simulink model "BlueROV2_Exp_Simu_NIF"  (R2023b)
settings: Solver=FixedStepAuto  StartTime=0.0  StopTime=120  FixedStep=dt  RelTol=1e-3
values from neighbouring files (symbols this model uses):
  Af = diag(ti)    [RM_param_AGF.m]
  Ballast_Force = Ballast_Compute(Ballast_Config)    [Integrate.m]    (also in init.m = Ballast_Term(Ballast_Config); init_NIF.m = [0; 0; Ballast_Term; 0]; init_NIF2.m = [0; 0; Ballast_Term; 0]; init_ODE.m)
  dt = 0.1    [Integrate.m]    (also in init.m; init_NIF.m; init_NIF2.m; init_ODE.m)
  Gamma = diag(omega_is)    [RM_param_AGF.m]
  Kd = [155; 355; 8985; 1205; 1205; 1]    [Integrate.m]    (also in init.m = [1; 1; 1; 1; 1; 1]; init_NIF.m; init_NIF2.m; init_ODE.m)
  Ki = [45; 45; 10; 96; 96; 1]    [Integrate.m]    (also in init.m = [1; 1; 1; 1; 1; 1]; init_NIF.m; init_NIF2.m; init_ODE.m)
  Kp = [255; 545; 7095; 2420; 2375; 1]    [Integrate.m]    (also in init.m = [1; 1; 1; 1; 1; 1]; init_NIF.m; init_NIF2.m; init_ODE.m)
  lower_limit = -upper_limit    (= -30)    [Integrate.m]    (also in init.m; init_NIF.m; init_NIF2.m; init_ODE.m)
  Omega = diag(2*omega_is.*zeta_is)    [RM_param_AGF.m]
  Param = BlueROV2_param()    [Integrate.m]    (also in init.m; init_NIF.m; init_NIF2.m; init_ODE.m)
  T_alloc = Thrust_Allocation()    [Integrate.m]    (also in init_NIF.m; init_NIF2.m; init_ODE.m; init_ballast_checking.m)
  T_alloc_ps = pinv(T_alloc' * T_alloc + lambda * eye(size(T_alloc, 2))) * T_alloc'    [Integrate.m]    (also in init_NIF.m; init_NIF2.m; init_ODE.m; init_ballast_checking.m)
  thrust_rate = 5    [Integrate.m]    (also in init.m; init_NIF.m; init_NIF2.m; init_ODE.m)
  upper_limit = 30    [Integrate.m]    (also in init.m; init_NIF.m; init_NIF2.m; init_ODE.m)
undefined symbols (not defined in the file or in its folder): model_val, Phi_ref, Psi_ref, resampled_time, Theta_ref, time_stamps_phi, time_stamps_psi, time_stamps_theta, time_stamps_x, time_stamps_y, time_stamps_z, time_val, X_ref, Y_ref, Z_ref
(part 2 of 2)

== matlab function BlueROV2_Exp_Simu_NIF/Real Model/BlueROV2/BLUEROV2 DYNAMIC/ROV_SYSTEM/DYNAMIC SOLVER/BlueROV2_EOM/Nonlinear Damping ==
  data: F_nld_o output; nu_b input; d_CB input; K_nl input
function F_nld_o = Nonlinear_Damping_forces(nu_b, d_CB, K_nl)
%% Nonlinear Damping Forces
% Velocity
u = nu_b(1);
v = nu_b(2);
w = nu_b(3);
p = nu_b(4);
q = nu_b(5);
r = nu_b(6);

% Distance from CB to CO
% Defined as d_CB

% Transformed Velocity
V_t_b = H_(-d_CB) * nu_b;  % 6DOF Velocity, expressed in CB

% Nonlinear Damping Matrix
NL_Damping_Coeff = diag(K_nl) * abs(V_t_b);

% Force
F_nld_o = -(H_(d_CB))' * diag(NL_Damping_Coeff) * V_t_b;

% For debugging
% F_nld_o = -diag(NL_Damping_Coeff) * nu_b;
% F_nld_o = zeros(6,1);
end

== matlab function BlueROV2_Exp_Simu_NIF/Real Model/Reference Model CIF/Heave/MATLAB Function ==
  data: t input; eta_ref output; resampled_model input; resampled_time input
function eta_ref = feedPositionReference(t, resampled_model, resampled_time)
    persistent positionData;
    persistent timeData;
    persistent currentIndex;
    
    % Load position and time data (you can load this data only once)
    if isempty(positionData)
        positionData = resampled_model; % Your position data
        timeData = resampled_time; % Your time data
        currentIndex = 1;
    end
    
    % Find the index corresponding to the current time
    while currentIndex < length(timeData) && timeData(currentIndex) < t
        currentIndex = currentIndex + 1;
    end
    
    % Output the position reference at the current time
    eta_ref = positionData(currentIndex);
end

== matlab function BlueROV2_Exp_Simu_NIF/Real Model/Reference Model CIF/Pitch/MATLAB Function ==
  data: t input; eta_ref output; resampled_model input; resampled_time input
function eta_ref = feedPositionReference(t, resampled_model, resampled_time)
    persistent positionData;
    persistent timeData;
    persistent currentIndex;
    
    % Load position and time data (you can load this data only once)
    if isempty(positionData)
        positionData = resampled_model; % Your position data
        timeData = resampled_time; % Your time data
        currentIndex = 1;
    end
    
    % Find the index corresponding to the current time
    while currentIndex < length(timeData) && timeData(currentIndex) < t
        currentIndex = currentIndex + 1;
    end
    
    % Output the position reference at the current time
    eta_ref = positionData(currentIndex);
end

== matlab function BlueROV2_Exp_Simu_NIF/Real Model/Reference Model CIF/Roll/MATLAB Function ==
  data: t input; eta_ref output; resampled_model input; resampled_time input
function eta_ref = feedPositionReference(t, resampled_model, resampled_time)
    persistent positionData;
    persistent timeData;
    persistent currentIndex;
    
    % Load position and time data (you can load this data only once)
    if isempty(positionData)
        positionData = resampled_model; % Your position data
        timeData = resampled_time; % Your time data
        currentIndex = 1;
    end
    
    % Find the index corresponding to the current time
    while currentIndex < length(timeData) && timeData(currentIndex) < t
        currentIndex = currentIndex + 1;
    end
    
    % Output the position reference at the current time
    eta_ref = positionData(currentIndex);
end

== matlab function BlueROV2_Exp_Simu_NIF/Real Model/BlueROV2/BLUEROV2 DYNAMIC/ROV_SYSTEM/DYNAMIC SOLVER/Rotation Matrix ==
  data: eta_n input; J_Theta_nb output
function J_Theta_nb = Transform_nb(eta_n)
%%%%%%%%%%%%%%%%%%%%%%%%%%%%%%%%%%%%%%%%%%%%%%%%%%%%%%%%%%%%%%%%%%%%%%%%%%%
% Command                                                                 %
%                                                                         %
% Compute the Jacobian from {b} to {n}                                    %
%                                                                         %
% For 6-DOF Equations:                                                    %
% [ndot = Jacobian(n_theta) * v]                                          %
% -ndot = velocity expressed in NED frame                                 %
% -n_theta = rotational part of position vector                           %
% - v = velocity expressed in Body frame                                  %
%                                                                         %
% Argument:                                                               %
% eta     : Input positional vector                                       %
%                                                                         %
% Created:      27.09.2023	Andreas Sitorus                               %
%                                                                         %
%%%%%%%%%%%%%%%%%%%%%%%%%%%%%%%%%%%%%%%%%%%%%%%%%%%%%%%%%%%%%%%%%%%%%%%%%%%
%% Get the orientation
phi = eta_n(4,1);       % Rolling angle
theta = eta_n(5,1);     % Pitching angle
psi = eta_n(6,1);       % Yaw angle

%% Linear Velocity Transformation Matrix
% Element
r11 = cos(psi) * cos(theta);
r12 = -sin(psi) * cos(phi) + cos(psi) * sin(theta) * sin(phi);
r13 = sin(psi) * sin(phi) + cos(psi) * cos(phi) * sin(theta);
r21 = sin(psi) * cos(theta);
r22 = cos(psi) * cos(phi) + sin(phi) * sin(theta) * sin(psi);
r23 = -cos(psi) * sin(phi) + sin(theta) * sin(psi) * cos(phi);
r31 = -sin(theta);
r32 = cos(theta) * sin(phi);
r33 = cos(theta) * cos(phi);

% Rotation Matrix (from {b} to {n})
R_Theta_nb = [r11 r12 r13;
              r21 r22 r23;
              r31 r32 r33];

%% Angular Velocity Transformation Matrix
% Element
t11 = 1;
t12 = sin(phi) * tan(theta);
t13 = cos(phi) * tan(theta);
t21 = 0;
t22 = cos(phi);
t23 = -sin(phi);
t31 = 0;
t32 = sin(phi) / cos(theta);
t33 = cos(phi) / cos(theta);

% Angular Velocity Rotation Matrix (from {b} to {n})
T_Theta_nb = [t11 t12 t13;
              t21 t22 t23;
              t31 t32 t33];

%% Jacobian
J_Theta_nb = [R_Theta_nb  zeros(3);
              zeros(3) T_Theta_nb];

end

== matlab function BlueROV2_Exp_Simu_NIF/Real Model/Reference Model CIF/Surge/MATLAB Function ==
  data: t input; eta_ref output; resampled_model input; resampled_time input
function eta_ref = feedPositionReference(t, resampled_model, resampled_time)
    persistent positionData;
    persistent timeData;
    persistent currentIndex;
    
    % Load position and time data (you can load this data only once)
    if isempty(positionData)
        positionData = resampled_model; % Your position data
        timeData = resampled_time; % Your time data
        currentIndex = 1;
    end
    
    % Find the index corresponding to the current time
    while currentIndex < length(timeData) && timeData(currentIndex) < t
        currentIndex = currentIndex + 1;
    end
    
    % Output the position reference at the current time
    eta_ref = positionData(currentIndex);
end

== matlab function BlueROV2_Exp_Simu_NIF/Real Model/Reference Model CIF/Sway/MATLAB Function ==
  data: t input; eta_ref output; resampled_model input; resampled_time input
function eta_ref = feedPositionReference(t, resampled_model, resampled_time)
    persistent positionData;
    persistent timeData;
    persistent currentIndex;
    
    % Load position and time data (you can load this data only once)
    if isempty(positionData)
        positionData = resampled_model; % Your position data
        timeData = resampled_time; % Your time data
        currentIndex = 1;
    end
    
    % Find the index corresponding to the current time
    while currentIndex < length(timeData) && timeData(currentIndex) < t
        currentIndex = currentIndex + 1;
    end
    
    % Output the position reference at the current time
    eta_ref = positionData(currentIndex);
end

== matlab function BlueROV2_Exp_Simu_NIF/Real Model/Reference Model CIF/Yaw/MATLAB Function ==
  data: t input; eta_ref output; resampled_model input; resampled_time input
function eta_ref = feedPositionReference(t, resampled_model, resampled_time)
    persistent positionData;
    persistent timeData;
    persistent currentIndex;
    
    % Load position and time data (you can load this data only once)
    if isempty(positionData)
        positionData = resampled_model; % Your position data
        timeData = resampled_time; % Your time data
        currentIndex = 1;
    end
    
    % Find the index corresponding to the current time
    while currentIndex < length(timeData) && timeData(currentIndex) < t
        currentIndex = currentIndex + 1;
    end
    
    % Output the position reference at the current time
    eta_ref = positionData(currentIndex);
end

== matlab function BlueROV2_Exp_Simu_NIF/For Estimation/BlueROV2/BLUEROV2 DYNAMIC/ROV_SYSTEM/DYNAMIC SOLVER/BlueROV2_EOM/Added Mass Coriolis-Centripetal ==
  data: nu_b input; F_Ca_o output; d_CB input; AM input
function F_Ca_o    = Coriolis_Centripetal_AM_Force(nu_b, d_CB, AM)
%% Coriolis-Centripetal Forces
% Velocity
u = nu_b(1);
v = nu_b(2);
w = nu_b(3);
p = nu_b(4);
q = nu_b(5);
r = nu_b(6);

% Distance from CB to CO
% Defined as d_CB

% Transformed Velocity
V_t_b = H_(-d_CB) * nu_b;  % 6DOF Velocity, expressed in CB

% Added Mass Coefficient
Xud = AM(1);
Yvd = AM(2);
Zwd = AM(3);
Kpd = AM(4);
Mqd = AM(5);
Nrd = AM(6);

% CC-Added Mass
% Described in Body frame, at Center of Buoyancy
Ca11 = zeros(3);
Ca12 = [0 -Zwd*w Yvd*v;
        Zwd*w 0 -Xud*u;
        -Yvd*v Xud*u 0];
Ca21 = Ca12;
Ca22 = [0 -Nrd*r Mqd*q;
        Nrd*r 0 -Kpd*p;
        -Mqd*q Kpd*p 0];

Ca = [Ca11 Ca12;
      Ca21 Ca22]; % Added mass Coriolis Force Matrix, at Center of Buoyancy

% Force
% F_Ca_o = (H_(d_CB))' * Ca * V_t_b;

% For debugging
% F_Ca_o = Ca * nu_b;
F_Ca_o = zeros(6,1);
end

== matlab function BlueROV2_Exp_Simu_NIF/For Estimation/BlueROV2/BLUEROV2 DYNAMIC/ROV_SYSTEM/DYNAMIC SOLVER/BlueROV2_EOM/Linear Damping ==
  data: F_ld_o output; nu_b input; d_CB input; K_l input
function F_ld_o  = Linear_Damping(nu_b, d_CB, K_l)
% %% Linear Damping Forces
% % Distance from CB to CO
% % Defined as d_CB

% Transformed Velocity
V_t_b = H_(-d_CB) * nu_b;  % 6DOF Velocity, expressed in CB

% Force
F_ld_o = -(H_(d_CB)) * diag(K_l) * V_t_b; 

% For debugging
% F_ld_o = -diag(L_Damping_Matrix) * nu_b; 
% F_ld_o = zeros(6,1); 
end

== matlab function BlueROV2_Exp_Simu_NIF/For Estimation/BlueROV2/BLUEROV2 DYNAMIC/ROV_SYSTEM/DYNAMIC SOLVER/BlueROV2_EOM/Nonlinear Damping ==
  data: F_nld_o output; nu_b input; d_CB input; K_nl input
function F_nld_o = Nonlinear_Damping_forces(nu_b, d_CB, K_nl)
%% Nonlinear Damping Forces
% Velocity
u = nu_b(1);
v = nu_b(2);
w = nu_b(3);
p = nu_b(4);
q = nu_b(5);
r = nu_b(6);

% Distance from CB to CO
% Defined as d_CB

% Transformed Velocity
V_t_b = H_(-d_CB) * nu_b;  % 6DOF Velocity, expressed in CB

% Nonlinear Damping Matrix
NL_Damping_Coeff = diag(K_nl) * abs(V_t_b);

% Force
F_nld_o = -(H_(d_CB))' * diag(NL_Damping_Coeff) * V_t_b;

% For debugging
% F_nld_o = -diag(NL_Damping_Coeff) * nu_b;
% F_nld_o = zeros(6,1);
end

== matlab function BlueROV2_Exp_Simu_NIF/For Estimation/BlueROV2/BLUEROV2 DYNAMIC/ROV_SYSTEM/DYNAMIC SOLVER/BlueROV2_EOM/Restoring Force ==
  data: eta_n input; F_r_o output; CG input; CB input; W input; B input
function F_r_o   = Restoring_Force(eta_n, CG, CB, W, B)
%% Restoring Forces
% Described in Body Frame, at Center of Gravity. ALREADY FOR THE LEFT HAND SIDE
% Orientation
phi = eta_n(4);
theta = eta_n(5);

% Gravity
xg = CG(1);
yg = CG(2);
zg = CG(3);

% Buoyancy
xb = CB(1);
yb = CB(2);
zb = CB(3);

% % Force
% Fg_n = [0; 0; W];
% Fb_n = -[0; 0; B];
% 
% F_r_o = -[Rot_bn(eta_n) * Fg_n + Rot_bn(eta_n) * Fb_n;
%          cross(CG, Rot_bn(eta_n) * Fg_n) + cross(CB, Rot_bn(eta_n) * Fb_n)];

% Force
F_r_o = [(W - B)*sin(theta);
         -(W - B)*cos(theta)*sin(phi);
         -(W - B)*cos(theta)*cos(phi);
         -(yg*W - yb*B)*cos(theta)*cos(phi) + (zg*W - zb*B)*cos(theta)*sin(phi);
         (zg*W - zb*B)*sin(theta) + (xg*W - xb*B)*cos(theta)*cos(phi);
         -(xg*W - xb*B)*cos(theta)*sin(phi) - (yg*W - yb*B)*sin(theta)];

% For debugging
% F_r_o = zeros(6,1);
end

== matlab function BlueROV2_Exp_Simu_NIF/Real Model/Controller (PID)/Transformation_bn Position ==
  data: phi input; J_Theta_bn output; theta input; psi input
function J_Theta_bn  = Transform_bn(phi, theta, psi)
%%%%%%%%%%%%%%%%%%%%%%%%%%%%%%%%%%%%%%%%%%%%%%%%%%%%%%%%%%%%%%%%%%%%%%%%%%%
% Command                                                                 %
%                                                                         %
% Compute the Jacobian inverse from {n} to {b}                            %
%                                                                         %
% For 6-DOF Equations:                                                    %
% [ndot = Jacobian(n_theta) * v]                                          %
% -ndot = velocity expressed in NED frame                                 %
% -n_theta = rotational part of position vector                           %
% - v = velocity expressed in Body frame                                  %
%                                                                         %
% Argument:                                                               %
% eta     : Input positional vector                                       %
%                                                                         %
% Created:      27.09.2023	Andreas Sitorus                               %
%                                                                         %
%%%%%%%%%%%%%%%%%%%%%%%%%%%%%%%%%%%%%%%%%%%%%%%%%%%%%%%%%%%%%%%%%%%%%%%%%%%
%% Get the orientation
% Phi   = Rolling angle
% Theta = Pitching angle
% Psi   = Yaw angle

%% Linear Velocity Transformation Matrix
% Element
r11 = cos(psi) * cos(theta);
r12 = cos(theta) * sin(psi);
r13 = -sin(theta);
r21 = cos(psi) * sin(phi) * sin(theta) - sin(psi) * cos(phi);
r22 = cos(phi) * cos(psi) + sin(phi) * sin(psi) * sin(theta);
r23 = cos(theta) * sin(phi);
r31 = sin(phi) * sin(psi) + cos(phi) * cos(psi) * sin(theta);
r32 = cos(phi) * sin(psi) * sin(theta) - cos(psi) * sin(phi);
r33 = cos(phi) * cos(theta);

% Rotation Matrix (from {n} to {b})
R_Theta_bn = [r11 r12 r13;
              r21 r22 r23;
              r31 r32 r33];

%% Angular Velocity Transformation Matrix
% Element
t11 = 1;
t12 = 0;
t13 = -sin(theta);
t21 = 0;
t22 = cos(phi);
t23 = cos(theta) * sin(phi);
t31 = 0;
t32 = -sin(phi);
t33 = cos(theta) * cos(phi);

% Angular Velocity Rotation Matrix (from {n} to {b})
T_Theta_bn = [t11 t12 t13;
              t21 t22 t23;
              t31 t32 t33];

%% Jacobian
J_Theta_bn = [R_Theta_bn  zeros(3);
               zeros(3) T_Theta_bn];
end

== matlab function BlueROV2_Exp_Simu_NIF/Real Model/Controller (PID)/Transformation_bn Velocity ==
  data: phi input; J_Theta_bn output; theta input; psi input
function J_Theta_bn  = Transform_bn(phi, theta, psi)
%%%%%%%%%%%%%%%%%%%%%%%%%%%%%%%%%%%%%%%%%%%%%%%%%%%%%%%%%%%%%%%%%%%%%%%%%%%
% Command                                                                 %
%                                                                         %
% Compute the Jacobian inverse from {n} to {b}                            %
%                                                                         %
% For 6-DOF Equations:                                                    %
% [ndot = Jacobian(n_theta) * v]                                          %
% -ndot = velocity expressed in NED frame                                 %
% -n_theta = rotational part of position vector                           %
% - v = velocity expressed in Body frame                                  %
%                                                                         %
% Argument:                                                               %
% eta     : Input positional vector                                       %
%                                                                         %
% Created:      27.09.2023	Andreas Sitorus                               %
%                                                                         %
%%%%%%%%%%%%%%%%%%%%%%%%%%%%%%%%%%%%%%%%%%%%%%%%%%%%%%%%%%%%%%%%%%%%%%%%%%%
%% Get the orientation
% Phi   = Rolling angle
% Theta = Pitching angle
% Psi   = Yaw angle

%% Linear Velocity Transformation Matrix
% Element
r11 = cos(psi) * cos(theta);
r12 = cos(theta) * sin(psi);
r13 = -sin(theta);
r21 = cos(psi) * sin(phi) * sin(theta) - sin(psi) * cos(phi);
r22 = cos(phi) * cos(psi) + sin(phi) * sin(psi) * sin(theta);
r23 = cos(theta) * sin(phi);
r31 = sin(phi) * sin(psi) + cos(phi) * cos(psi) * sin(theta);
r32 = cos(phi) * sin(psi) * sin(theta) - cos(psi) * sin(phi);
r33 = cos(phi) * cos(theta);

% Rotation Matrix (from {n} to {b})
R_Theta_bn = [r11 r12 r13;
              r21 r22 r23;
              r31 r32 r33];

%% Angular Velocity Transformation Matrix
% Element
t11 = 1;
t12 = 0;
t13 = -sin(theta);
t21 = 0;
t22 = cos(phi);
t23 = cos(theta) * sin(phi);
t31 = 0;
t32 = -sin(phi);
t33 = cos(theta) * cos(phi);

% Angular Velocity Rotation Matrix (from {n} to {b})
T_Theta_bn = [t11 t12 t13;
              t21 t22 t23;
              t31 t32 t33];

%% Jacobian
J_Theta_bn = [R_Theta_bn  zeros(3);
               zeros(3) T_Theta_bn];
end

== matlab function BlueROV2_Exp_Simu_NIF/For Estimation/BlueROV2/BLUEROV2 DYNAMIC/ROV_SYSTEM/DYNAMIC SOLVER/BlueROV2_EOM/Rigid Body Coriolis-Centripetal ==
  data: nu_b input; F_Crb_o output; d_CG input; MOI input; m input
function F_Crb_o    = Coriolis_Centripetal_RB_Force(nu_b, d_CG, MOI, m)
%% Coriolis-Centripetal Forces
% Velocity
u = nu_b(1);
v = nu_b(2);
w = nu_b(3);
p = nu_b(4);
q = nu_b(5);
r = nu_b(6);

% Distance from CG to CO
% Defined as d_CG

% Transformed Velocity
V_t_g = H_(-d_CG) * nu_b;  % 6DOF Velocity, expressed in CG

% MOI
Ixx = MOI(1);
Iyy = MOI(2);
Izz = MOI(3);

% CC-Rigid Body
% Described in Body frame, at Center of Gravity

Crb11 = zeros(3); 
Crb12 = [0 m*w -m*v;
         -m*w 0 m*u;
         m*v -m*u 0];
Crb21 = Crb12;
Crb22 = [0 -Izz*r -Iyy*q;
         Izz*r 0 Ixx*p;
         Iyy*q -Ixx*p 0];

Crb = [Crb11 Crb12;
       Crb21 Crb22]; % Rigid Body Coriolis Force Matrix, at Center of Gravity

% Force
% F_Crb_o = (H_(d_CG))' * Crb * V_t_g;

% For debugging
% F_Crb_o = Crb * nu_b;
F_Crb_o = zeros(6,1);
end

== matlab function BlueROV2_Exp_Simu_NIF/For Estimation/BlueROV2/BLUEROV2 DYNAMIC/ROV_SYSTEM/DYNAMIC SOLVER/Rotation Matrix ==
  data: eta_n input; J_Theta_nb output
function J_Theta_nb = Transform_nb(eta_n)
%%%%%%%%%%%%%%%%%%%%%%%%%%%%%%%%%%%%%%%%%%%%%%%%%%%%%%%%%%%%%%%%%%%%%%%%%%%
% Command                                                                 %
%                                                                         %
% Compute the Jacobian from {b} to {n}                                    %
%                                                                         %
% For 6-DOF Equations:                                                    %
% [ndot = Jacobian(n_theta) * v]                                          %
% -ndot = velocity expressed in NED frame                                 %
% -n_theta = rotational part of position vector                           %
% - v = velocity expressed in Body frame                                  %
%                                                                         %
% Argument:                                                               %
% eta     : Input positional vector                                       %
%                                                                         %
% Created:      27.09.2023	Andreas Sitorus                               %
%                                                                         %
%%%%%%%%%%%%%%%%%%%%%%%%%%%%%%%%%%%%%%%%%%%%%%%%%%%%%%%%%%%%%%%%%%%%%%%%%%%
%% Get the orientation
phi = eta_n(4,1);       % Rolling angle
theta = eta_n(5,1);     % Pitching angle
psi = eta_n(6,1);       % Yaw angle

%% Linear Velocity Transformation Matrix
% Element
r11 = cos(psi) * cos(theta);
r12 = -sin(psi) * cos(phi) + cos(psi) * sin(theta) * sin(phi);
r13 = sin(psi) * sin(phi) + cos(psi) * cos(phi) * sin(theta);
r21 = sin(psi) * cos(theta);
r22 = cos(psi) * cos(phi) + sin(phi) * sin(theta) * sin(psi);
r23 = -cos(psi) * sin(phi) + sin(theta) * sin(psi) * cos(phi);
r31 = -sin(theta);
r32 = cos(theta) * sin(phi);
r33 = cos(theta) * cos(phi);

% Rotation Matrix (from {b} to {n})
R_Theta_nb = [r11 r12 r13;
              r21 r22 r23;
              r31 r32 r33];

%% Angular Velocity Transformation Matrix
% Element
t11 = 1;
t12 = sin(phi) * tan(theta);
t13 = cos(phi) * tan(theta);
t21 = 0;
t22 = cos(phi);
t23 = -sin(phi);
t31 = 0;
t32 = sin(phi) / cos(theta);
t33 = cos(phi) / cos(theta);

% Angular Velocity Rotation Matrix (from {b} to {n})
T_Theta_nb = [t11 t12 t13;
              t21 t22 t23;
              t31 t32 t33];

%% Jacobian
J_Theta_nb = [R_Theta_nb  zeros(3);
              zeros(3) T_Theta_nb];

end
